simulink model "ValidaCabeceo"  (R2024a)
settings: Solver=VariableStepAuto  StartTime=0.0  StopTime=8  MaxStep=0.01  RelTol=1e-3
values from neighbouring files (symbols this model uses):
  A = Kp*((1+((2*bheta*Td)/(h_digitalizacion))))    [disenCabeceo.m]
  B = Kp*((1-((2*bheta*Td)/(h_digitalizacion))))    [disenCabeceo.m]
  C = Kp*((1+((2*Td)/(h_digitalizacion))))    [disenCabeceo.m]
  D = Kp*((1-((2*Td)/(h_digitalizacion))))    [disenCabeceo.m]
  G_den = den    [disenCabeceo.m]
  G_num = num    [disenCabeceo.m]
  h_digitalizacion = (2*pi)/(20*Wn)    [disenCabeceo.m]
  Mp = 10/100    (= 0.1)    [disenCabeceo.m]
libraries: simulink x1
settings Model: Creator=david  LastModifiedBy=david

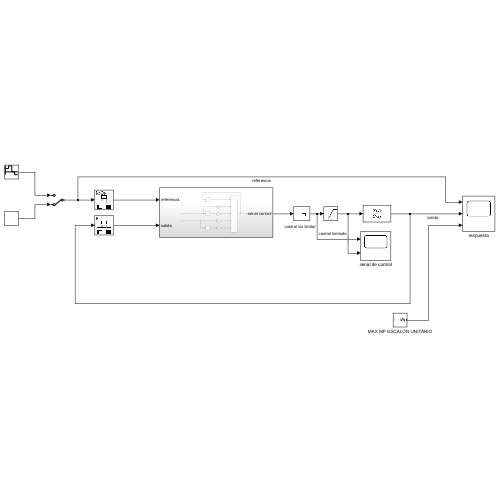
[thumbnail: Simulink's stored preview of the top-level diagram]
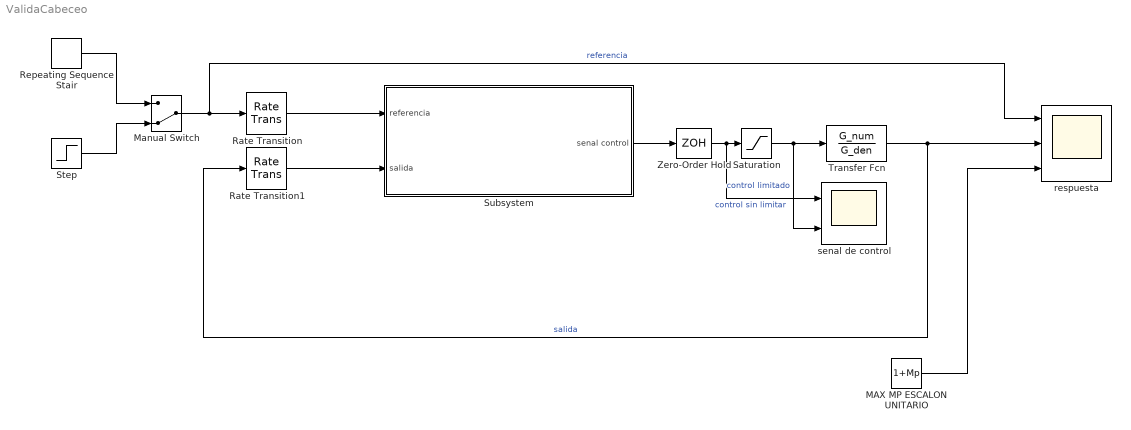
== system ValidaCabeceo ==
  MAX MP ESCALON UNITARIO : Constant  Value=1+Mp
  Manual Switch : ManualSwitch  CurrentSetting=0
  Rate Transition : RateTransition  Integrity=off  OutPortSampleTime=h_digitalizacion
  Rate Transition1 : RateTransition  Integrity=off  OutPortSampleTime=h_digitalizacion
  Repeating Sequence Stair : simulink/Sources/Repeating Sequence Stair  OutValues=[pi/4 pi/2 0 -pi/4].'  tsamp=2  OutMin=[]  OutMax=[]  OutDataTypeStr=double  OutputDataTypeScalingMode=double  OutDataType=fixdt(0,8)  ConRadixGroup=Best Precision: Vector-wise  OutScaling=2^-12
  Saturation : Saturate  UpperLimit=10  LowerLimit=-10
  Step : Step  SampleTime=h_digitalizacion
  Subsystem : Subsystem
  Transfer Fcn : TransferFcn  Numerator=G_num  Denominator=G_den
  Zero-Order Hold : ZeroOrderHold  SampleTime=h_digitalizacion
  respuesta : Scope  NumInputPorts=3
  senal de control : Scope  NumInputPorts=2
  wires:
  Repeating Sequence Stair/1 -> Manual Switch/1
  Step/1 -> Manual Switch/2
  Rate Transition/1 -> Subsystem/1(referencia)
  Rate Transition1/1 -> Subsystem/2(salida)
  Manual Switch/1 -> Rate Transition/1, respuesta/1  "referencia"
  Zero-Order Hold/1 -> senal de control/1, Saturation/1  "control sin limitar"
  Subsystem/1(senal control) -> Zero-Order Hold/1
  Saturation/1 -> senal de control/2, Transfer Fcn/1  "control limitado"
  Transfer Fcn/1 -> Rate Transition1/1, respuesta/2  "salida"
  MAX MP ESCALON UNITARIO/1 -> respuesta/3

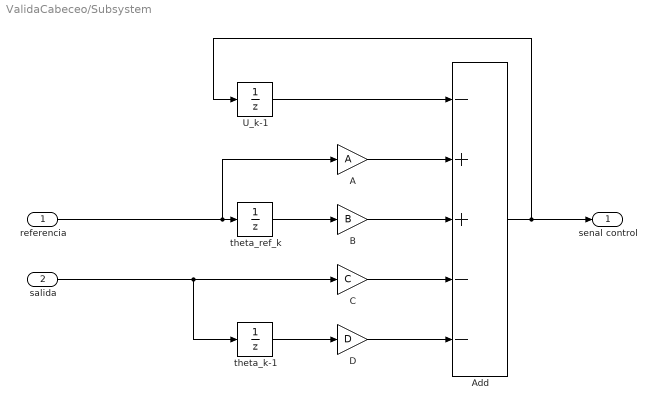
== system ValidaCabeceo/Subsystem ==
  referencia : Inport
  salida : Inport  Port=2
  A : Gain  Gain=A
  Add : Sum  Inputs=-++--
  B : Gain  Gain=B
  C : Gain  Gain=C
  D : Gain  Gain=D
  U_k-1 : UnitDelay  SampleTime=h_digitalizacion  HasFrameUpgradeWarning=on
  theta_k-1 : UnitDelay  SampleTime=h_digitalizacion  HasFrameUpgradeWarning=on
  theta_ref_k : UnitDelay  SampleTime=h_digitalizacion  HasFrameUpgradeWarning=on
  senal control : Outport
  wires:
  A/1 -> Add/2
  theta_ref_k/1 -> B/1
  C/1 -> Add/4
  B/1 -> Add/3
  D/1 -> Add/5
  U_k-1/1 -> Add/1
  referencia/1 -> A/1, theta_ref_k/1
  theta_k-1/1 -> D/1
  salida/1 -> theta_k-1/1, C/1
  Add/1 -> senal control/1, U_k-1/1
